simulink model "pe_marine_electrical_system"  (R2018b)
settings: Solver=ode23t  StartTime=0.0  StopTime=70  MaxStep=1e-3  RelTol=1e-3  AbsTol=1e-3
undefined symbols (not defined in the file): pe
libraries: fl_lib x41, pe_lib x25, nesl_utility x14, peSmAC1C x2, simulink x2
Description:
  | Marine Full Electric Propulsion Power System
  | 
  | This example shows a representative marine half-ship electrical power system with
  | base load, hotel load, bow thrusters and electric propulsion.
  | 
  | The principal components of the system are:
  | *) 30 MVA Gas Turbine, Round Rotor Alternator
  | *) 5 MVA Diesel Generator, Salient Pole Alternator
  | *) 11.5 MVA Base Load
  | *) 6 MVA Switched Hotel Load
  | *) 20 MVA Average-Value Propulsion Rectifier
  | *) 1 MVA Direct Online Start, Squirrel Cage Bow Thrusters
  | 
  | The sequence of events during the simulation is:
  | *) 10 seconds - Hotel Load disconnected
  | *) 20 seconds - Propulsion begins ramping up
  | *) 30 seconds - Full power ahead
  | *) 40 seconds - Propulsion begins ramping down
  | *) 50 seconds - Bow Thrusters start up
  | *) 60 seconds - Hotel Load connected
  | 
  | To view full results, run the simulation, and enter at the MATLAB command
  | prompt: sscexplore(pe_marine_electrical_system_simlog)
  | 
  | Copyright 2014-2017 The MathWorks, Inc.
settings Model: Creator=The MathWorks, Inc.  LastModifiedBy=hood000j
settings SolverCC: AutoScaleAbsTol=off  MaxConsecutiveMinStep=5
settings DataIOCC: LimitDataPoints=on  SaveFormat=Array
settings OptimizationCC: BlockReduction=off  BooleanDataType=off  LifeSpan=inf
settings DebuggingCC: SaveWithParameterizedLinksMsg=none  UnderspecifiedInitializationDetection=Classic  MergeDetectMultiDrivingBlocksExec=none  SignalResolutionControl=TryResolveAllWithWarning  AllowSymbolicDim=off  LibraryContextMissingDiagnostic=none  StrictBusMsg=ErrorOnBusTreatedAsVector  SFUnexpectedBacktrackingDiag=warning  SFNoUnconditionalDefaultTransitionDiag=warning  SFExecutionAtInitializationDiag=none
settings HardwareCC: ProdBitPerPointer=32  ProdBitPerSizeT=32  ProdBitPerPtrDiffT=32  ProdLargestAtomicFloat=None  ProdIntDivRoundTo=Undefined  ProdEndianess=Unspecified  ProdWordSize=32  ProdHWDeviceType=32-bit Generic  TargetUnknown=on
settings ModelReferenceCC: PropagateSignalLabelsOutOfModel=off
settings SFSimCC: SimUseLocalCustomCode=off
settings RTWCC: RTWUseLocalCustomCode=off
settings CodeAppCC: StateflowObjectComments=on
settings GRTTargetCC: TargetLangStandard=C89/C90 (ANSI)  GeneratePreprocessorConditionals=Disable all
settings ConfigComp: CovMetricSettings=dw  CovHtmlReporting=on  CovSaveCumulativeToWorkspaceVar=on  CovSaveSingleToWorkspaceVar=on  CovExternalEMLEnable=off  CovSFcnEnable=off
settings SimscapeCC: SimscapeLogType=local  SimscapeLogName=pe_marine_electrical_system_simlog  SimscapeLogLimitData=off

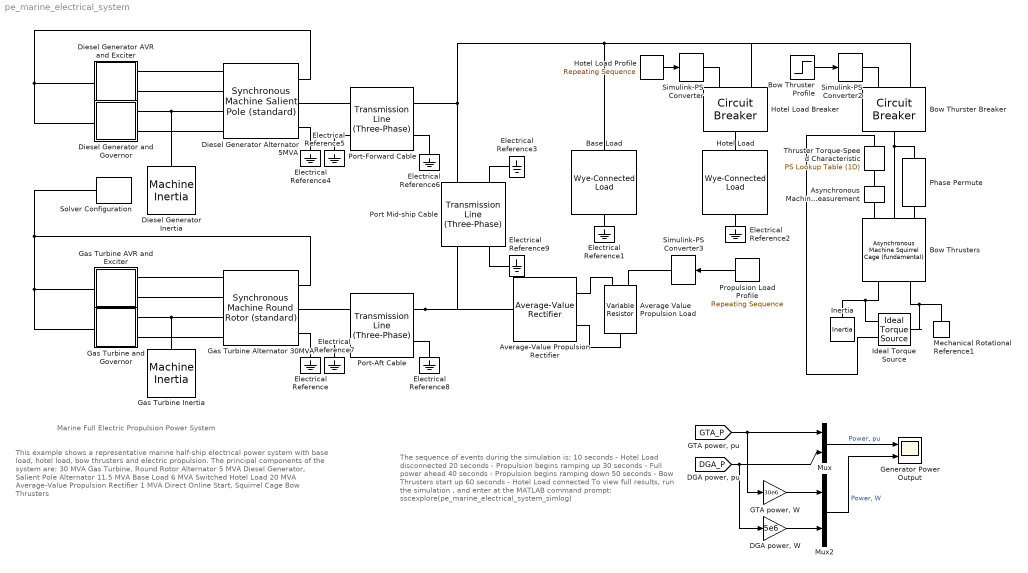
== system pe_marine_electrical_system ==
  note: The sequence of events during the simulation is:
      | 10 seconds - Hotel Load disconnected
      | 20 seconds - Propulsion begins ramping up
      | 30 seconds - Full power ahead
      | 40 seconds - Propulsion begins ramping down
      | 50 seconds - Bow Thrusters start up
      | 60 seconds - Hotel Load connected
      | To view full results, run the simulation , and enter at the MATLAB command
      | prompt: sscexplore(pe_marine_electrical_system_simlog)
  note: Marine Full Electric Propulsion Power System
  note: This example shows a representative marine half-ship electrical power system with
      | base load, hotel load, bow thrusters and electric propulsion.
      | The principal components of the system are:
      | 30 MVA Gas Turbine, Round Rotor Alternator
      | 5 MVA Diesel Generator, Salient Pole Alternator
      | 11.5 MVA Base Load
      | 6 MVA Switched Hotel Load
      | 20 MVA Average-Value Propulsion Rectifier
      | 1 MVA Direct Online Start, Squirrel Cage Bow Thrusters
  Asynchronous Machine Measurement : pe_lib/Machines/Asynchronous Machine Measurement  output_idx=2
      settings: SourceProductName=Simscape Power Systems  SourceProductBaseCode=PS  LogSimulationData=on
  Average Value Propulsion Load : fl_lib/Electrical/Electrical Elements/Variable Resistor  Rmin=0 Ohm  i_specify=off  i_priority=High  i=0 A  i_nominal_specify=off  i_nominal_unit=A  i_nominal_value=1  v_specify=off  v_priority=High  v=0 V  v_nominal_specify=off  v_nominal_unit=V  v_nominal_value=1
      settings: LogSimulationData=on
  Average-Value Propulsion Rectifier : pe_lib/Semiconductors/Average-Value Rectifier  VRated=4160 V  Pfixed=50e3 W
      settings: SourceProductName=Simscape Power Systems  SourceProductBaseCode=PS  LogSimulationData=on
  Base Load : pe_lib/Passive Devices/Wye-Connected Load  parameterization=2  component_structure=1  component_structure_PQ=4  R=1 Ohm  L=0.001 H  C=1e-6 F  IL0=[ 0 0 0 ] A  VC0=[ 0 0 0 ] V  R_parasitic=1e-6 Ohm  G_parasitic=1e-6 1/Ohm  VRated=4160 V  FRated=60 Hz  P=11.5e6 W  Qpos=700e3 V*A  Qneg=-100 V*A  Vmag0=4160 V  Vang0=0 deg  Freq0=60 Hz  R_parasitic_PQ=1e-6 Ohm  G_parasitic_PQ=1e-6 1/Ohm
      settings: SourceProductName=Simscape Power Systems  SourceProductBaseCode=PS  LogSimulationData=on
  Bow Thruster Profile : Step  Time=50  Before=1  After=0  SampleTime=0
  Bow Thrusters : pe_lib/Machines/Asynchronous Machine (Squirrel Cage)/Asynchronous Machine Squirrel Cage (fundamental)  SRated=1e6 V*A  VRated=4160 V  FRated=60 Hz  nPolePairs=5  squirrel_cage=pe.machines.asm_squirrel_cage.squirrelcage.Single  zero_sequence=pe.enum.park.zerosequence.include  Rs=0.0258  Lls=0.0930  Rrd=0.0145  Llrd=0.0424  Rrd1=0.0290  Llrd1=0.0848  Rrd2=0.0290  Llrd2=0.0848  Lm=1.7562  L0=0.0930  saturation_option=0  saturation_i=[0, .176, .396, .792, 1.1, 1.496, 2.2, 2.992, 4.18, 5.28]  saturation_v=[0, .2309, .4041, .5196, .5774, .6351, .6928, .7506, .8083, .866]  connection_option=int32(pe.Connection.delta)  param_option=pe.Parameterization.pu  angular_position_specify=off  angular_position_priority=None  angular_position=0 deg  angular_position_nominal_specify=off  angular_position_nominal_unit=deg  angular_position_nominal_value=1  pu_psids_specify=off  pu_psids_priority=None  pu_psids=0  pu_psids_nominal_specify=off  pu_psids_nominal_unit=1  pu_psids_nominal_value=1  pu_psiqs_specify=off  pu_psiqs_priority=None  pu_psiqs=0  pu_psiqs_nominal_specify=off  pu_psiqs_nominal_unit=1  pu_psiqs_nominal_value=1  pu_psi0s_specify=off  pu_psi0s_priority=None  pu_psi0s=0  pu_psi0s_nominal_specify=off  pu_psi0s_nominal_unit=1  pu_psi0s_nominal_value=1
      settings: SourceProductName=Simscape Power Systems  SourceProductBaseCode=PS  LogSimulationData=on
  Bow Thurster Breaker : pe_lib/Switches & Breakers/Circuit Breaker  R_closed=0.001 Ohm  G_open=1e-4 1/Ohm  threshold=0.5 V
      settings: SourceProductName=Simscape Power Systems  SourceProductBaseCode=PS  LogSimulationData=on
  "DGA power, W" : Gain  Gain=5e6
  Diesel Generator AVR and Exciter : Subsystem
  Diesel Generator Alternator 5MVA : pe_lib/Machines/Synchronous Machine (Salient Pole)/Synchronous Machine Salient Pole (standard)  SRated=5e6 V*A  VRated=4160 V  FRated=60 Hz  nPolePairs=4  fieldCircuitParameterization_option=2  baseEfd=216.54 V  baseIfd=50 A  zero_sequence=pe.enum.park.zerosequence.include  Ra=0.011  Xl=0.15  Xd=1.05  Xq=0.7  X0=0.15  Xdd=0.35  Xddd=0.25  Xqdd=0.325  d_option=1  Td0d=5.25 s  Tdd=1.75 s  Td0dd=0.03 s  Tddd=0.0214 s  q_option=1  Tq0dd=0.05 s  Tqdd=0.0232 s  saturation_option=0  axes_param=pe.enum.rotorangle.daxis  saturation_ifd=[0.00, 0.48, 0.76, 1.38, 1.79]  saturation_Vag=[0.00, 0.43, 0.59, 0.71, 0.76]  initialization_option=2  angular_position0=0 deg  pu_psid0=0  pu_psiq0=0  pu_psi00=0  pu_psifd0=0  pu_psi1d0=0  pu_psi1q0=0  Vmag0=4160 V  Vang0=0 deg  Pt0=2.5e6 V*A  Qt0=100e3 V*A  connection_option=int32(pe.Connection.wye)  num_q_dampers=1  rotor_offset=-pi / 2 rad  Xmin=1e-9
      settings: SourceProductName=Simscape Power Systems  SourceProductBaseCode=PS  LogSimulationData=on
  Diesel Generator Inertia : pe_lib/Machines/Machine Inertia  SRated=5e6 V*A  FRated=60 Hz  nPolePairs=4  inertia_option=2  J=27548 kg*m^2  H=3.525 s*W/V/A  damper_option=2  D=39.0509 N*m/(rad/s)  pu_D=0.01  initialization_option=2  fMechanical0=60 Hz  fElectrical0=60 Hz
      settings: SourceProductName=Simscape Power Systems  SourceProductBaseCode=PS  LogSimulationData=on
  Diesel Generator and Governor : Subsystem  mask(Governor and Prime Mover){pu_speed_reference=0.998, droop_percentage=5, pu_load_reference_setpoint=0.5, T_G=0.2, T_DG=0.3, base_torque=53051.6, pu_torque0=0.502754}
      mask prompts: pu_speed_reference "Speed reference, (pu)"; droop_percentage "Percentage droop, (%)"; pu_load_reference_setpoint "Load reference setpoint, (pu)"; T_G "Time constant of governor, (s)"; T_DG "Time constant of diesel generator, (s)"; base_torque "Base torque, (N*m)"; pu_torque0 "Initial torque, (pu)"
      mask help:
      | Implements a synchronous machine governor and prime mover. The prime mover is a diesel generator.
      |
      | The input to the block is a per-unit synchronous machine measurement vector.
      |
      | R and C are mechanical rotational ports.
  Electrical Reference{,1..9} (10 alike) : fl_lib/Electrical/Electrical Elements/Electrical Reference
  "GTA power, W" : Gain  Gain=30e6
  Gas Turbine AVR and Exciter : Subsystem
  Gas Turbine Inertia : pe_lib/Machines/Machine Inertia  SRated=30e6 V*A  FRated=60 Hz  nPolePairs=1  inertia_option=2  J=27548 kg*m^2  H=2.525 s*W/V/A  damper_option=2  D=39.0509 N*m/(rad/s)  pu_D=0.01  initialization_option=2  fMechanical0=60 Hz  fElectrical0=60 Hz
      settings: SourceProductName=Simscape Power Systems  SourceProductBaseCode=PS  LogSimulationData=on
  "Gas Turbine and Governor " : Subsystem  mask(Governor and Prime Mover){pu_speed_reference=0.998, droop_percentage=5, pu_load_reference_setpoint=0.5, T_G=0.1, T_GT=0.2, base_torque=79577.5, pu_torque0=0.500751}
      mask prompts: pu_speed_reference "Speed reference, (pu)"; droop_percentage "Percentage droop, (%)"; pu_load_reference_setpoint "Load reference setpoint, (pu)"; T_G "Time constant of governor, (s)"; T_GT "Time constant of gas turbine, (s)"; base_torque "Base torque, (N*m)"; pu_torque0 "Initial torque, (pu)"
      mask help:
      | Implements a synchronous machine governor and prime mover. The prime mover is a gas turbine.
      |
      | The input to the block is a per-unit synchronous machine measurement vector.
      |
      | R and C are mechanical rotational ports.
  Gas Turbine Alternator 30MVA : pe_lib/Machines/Synchronous Machine (Round Rotor)/Synchronous Machine Round Rotor (standard)  SRated=30e6 V*A  VRated=4160 V  FRated=60 Hz  nPolePairs=1  fieldCircuitParameterization_option=2  baseEfd=92.95 V  baseIfd=200 A  zero_sequence=pe.enum.park.zerosequence.include  Ra=0.003  Xl=0.15  Xd=1.81  Xq=1.76  X0=0.15  Xdd=0.3  Xqd=0.65  Xddd=0.23  Xqdd=0.25  d_option=1  Td0d=8 s  Tdd=1.3260 s  Td0dd=0.03 s  Tddd=0.0230 s  q_option=1  Tq0d=1 s  Tqd=0.3693 s  Tq0dd=0.07 s  Tqdd=0.0269 s  saturation_option=0  axes_param=pe.enum.rotorangle.daxis  saturation_ifd=[0.00, 0.48, 0.76, 1.38, 1.79]  saturation_Vag=[0.00, 0.80, 1.08, 1.31, 1.40]  initialization_option=2  angular_position0=0 deg  pu_psid0=0  pu_psiq0=0  pu_psi00=0  pu_psifd0=0  pu_psi1d0=0  pu_psi1q0=0  pu_psi2q0=0  Vmag0=4160 V  Vang0=0 deg  Pt0=15e6 V*A  Qt0=600e3 V*A  connection_option=int32(pe.Connection.wye)  num_q_dampers=2  rotor_offset=-pi / 2 rad  Xmin=1e-9
      settings: SourceProductName=Simscape Power Systems  SourceProductBaseCode=PS  LogSimulationData=on
  Generator Power Output : Scope  NumInputPorts=2
  Hotel Load : pe_lib/Passive Devices/Wye-Connected Load  parameterization=2  component_structure=1  component_structure_PQ=1  R=1 Ohm  L=0.001 H  C=1e-6 F  IL0=[ 0 0 0 ] A  VC0=[ 0 0 0 ] V  R_parasitic=1e-6 Ohm  G_parasitic=1e-6 1/Ohm  VRated=4160 V  FRated=60 Hz  P=6e6 W  Qpos=10e6 V*A  Qneg=-100 V*A  Vmag0=2.4e+4 V  Vang0=0 deg  Freq0=60 Hz  R_parasitic_PQ=1e-6 Ohm  G_parasitic_PQ=1e-6 1/Ohm
      settings: SourceProductName=Simscape Power Systems  SourceProductBaseCode=PS  LogSimulationData=on
  Hotel Load Breaker : pe_lib/Switches & Breakers/Circuit Breaker  R_closed=0.001 Ohm  G_open=1e-4 1/Ohm  threshold=0.5 V
      settings: SourceProductName=Simscape Power Systems  SourceProductBaseCode=PS  LogSimulationData=on
  Hotel Load Profile : simulink/Sources/Repeating Sequence  rep_seq_t=[0 9.99 10 59.9 60 100]  rep_seq_y=[0 0 1 1 0 0]
  Ideal Torque Source : fl_lib/Mechanical/Mechanical Sources/Ideal Torque Source
      settings: LogSimulationData=on
  Inertia : fl_lib/Mechanical/Rotational Elements/Inertia  inertia=1000 kg*m^2  w_specify=off  w_priority=High  w=0 rad/s  w_nominal_specify=off  w_nominal_unit=rad/s  w_nominal_value=1  t_specify=off  t_priority=High  t=0 N*m  t_nominal_specify=off  t_nominal_unit=N*m  t_nominal_value=1
      settings: LogSimulationData=on
  Mechanical Rotational Reference1 : fl_lib/Mechanical/Rotational Elements/Mechanical Rotational Reference
  Mux : Mux  Inputs=2
  Mux2 : Mux  Inputs=2
  Phase Permute : pe_lib/Connections/Phase Permute
      settings: SourceProductName=Simscape Power Systems  SourceProductBaseCode=PS  LogSimulationData=on
  Port Mid-ship Cable : pe_lib/Passive Devices/Transmission Line (Three-Phase)  length=0.2 km  R=0.02 Ohm/km  L=0.5 mH/km  M=0.1 mH/km  Cl=0.3 uF/km  Cg=0 uF/km  Rm=0 Ohm/km  N=1  R_parasitic=1e-6 Ohm  G_parasitic=1e-6 1/Ohm
      settings: SourceProductName=Simscape Power Systems  SourceProductBaseCode=PS  LogSimulationData=on
  Port-Aft Cable : pe_lib/Passive Devices/Transmission Line (Three-Phase)  length=0.1 km  R=0.02 Ohm/km  L=0.5 mH/km  M=0.1 mH/km  Cl=0.3 uF/km  Cg=0 uF/km  Rm=0 Ohm/km  N=1  R_parasitic=1e-6 Ohm  G_parasitic=1e-6 1/Ohm
      settings: SourceProductName=Simscape Power Systems  SourceProductBaseCode=PS  LogSimulationData=on
  Port-Forward Cable : pe_lib/Passive Devices/Transmission Line (Three-Phase)  length=0.1 km  R=0.02 Ohm/km  L=0.5 mH/km  M=0.1 mH/km  Cl=0.3 uF/km  Cg=0 uF/km  Rm=0 Ohm/km  N=1  R_parasitic=1e-6 Ohm  G_parasitic=1e-6 1/Ohm
      settings: SourceProductName=Simscape Power Systems  SourceProductBaseCode=PS  LogSimulationData=on
  Propulsion Load Profile : simulink/Sources/Repeating Sequence  rep_seq_t=[0 20 27 30 40 43 50 100]  rep_seq_y=[100 100 10 2 2 10 100 100]
  Simulink-PS Converter : nesl_utility/Simulink-PS Converter  PhysicalDomain=network_engine_domain  SubClassName=ps_input  LeftPortType=input  RightPortType=output  PseudoPeriodic=off  Frequencies=[]  NoiseDistribution=none  NoiseParameters=[]  Unit=1  AffineConversion=off  FilteringAndDerivatives=zero  SimscapeFilterOrder=1  InputFilterTimeConstant=0.001  UdotUserProvided=1
  Simulink-PS Converter2 : nesl_utility/Simulink-PS Converter  PhysicalDomain=network_engine_domain  SubClassName=ps_input  LeftPortType=input  RightPortType=output  PseudoPeriodic=off  Frequencies=[]  NoiseDistribution=none  NoiseParameters=[]  Unit=1  AffineConversion=off  FilteringAndDerivatives=zero  SimscapeFilterOrder=1  InputFilterTimeConstant=0.001  UdotUserProvided=1
  Simulink-PS Converter3 : nesl_utility/Simulink-PS Converter  PhysicalDomain=network_engine_domain  SubClassName=ps_input  LeftPortType=input  RightPortType=output  PseudoPeriodic=off  Frequencies=[]  NoiseDistribution=none  NoiseParameters=[]  Unit=1  AffineConversion=off  FilteringAndDerivatives=zero  SimscapeFilterOrder=1  InputFilterTimeConstant=0.001  UdotUserProvided=1
  Solver Configuration : nesl_utility/Solver Configuration  PhysicalDomain=network_engine_domain  SubClassName=solver  LeftPortType=input  RightPortType=generic  Tones=[]  Harmonics=[]  SimulateNoise=off  Profile=off  UseLocalSampling=off  EnableSwitchedLinearOptims=on  FrequencyDomain=off  UseCCode=off  RelTol=0.001  AbsTol=1e-06  MinStep=1e-09  ToWorkspace=off  RevertToSquareIcSolve=off  NumHomotopyIterations=100  PhasorMode=off  PhasorModeNumHarmonics=1  DoDC=off  ResidualTolerance=1e-09  UseLocalSolver=on  LocalSolverChoice=NE_BACKWARD_EULER_ADVANCER  LocalSolverSampleTime=1e-3  DoFixedCost=on  MaxNonlinIter=3  MaxModeIter=2  LinearAlgebra=auto  EquationFormulation=NE_TIME_EF  DelaysMemoryBudget=1024  AutomaticFiltering=on  FilteringTimeConstant=0.001  PartitionStorageMethod=AS_NEEDED  PartitionMemoryBudget=1024
  Thruster Torque-Speed Characteristic : fl_lib/Physical Signals/Lookup Tables/PS Lookup Table (1D)  x=[0:0.1:2]  f=13262.9.*[0:0.1:2].^2  interp_method=2  extrap_method=1
      settings: SourceProductName=Simscape  SourceProductBaseCode=SS  LogSimulationData=on
  wires:
  Hotel Load Profile/1 -> Simulink-PS Converter/1
  Bow Thruster Profile/1 -> Simulink-PS Converter2/1
  Propulsion Load Profile/1 -> Simulink-PS Converter3/1
  [GTA_P] -> Mux/1, "GTA power, W"/1
  [DGA_P] -> Mux/2, "DGA power, W"/1
  Mux/1 -> Generator Power Output/1  "Power, pu"
  "GTA power, W"/1 -> Mux2/1
  "DGA power, W"/1 -> Mux2/2
  Mux2/1 -> Generator Power Output/2  "Power, W"
  connections:
  Electrical Reference1/LConn1 -- Base Load/RConn1
  Port-Aft Cable/RConn1 -- Port Mid-ship Cable/RConn1 -- Average-Value Propulsion Rectifier/LConn1
  Gas Turbine AVR and Exciter/RConn1 -- Gas Turbine Alternator 30MVA/LConn1
  Gas Turbine Alternator 30MVA/RConn1 -- "Gas Turbine and Governor "/LConn1 -- Gas Turbine AVR and Exciter/LConn1 -- Solver Configuration/RConn1
  Gas Turbine AVR and Exciter/RConn2 -- Gas Turbine Alternator 30MVA/LConn2
  Gas Turbine Alternator 30MVA/RConn3 -- Electrical Reference/LConn1
  "Gas Turbine and Governor "/RConn2 -- Gas Turbine Alternator 30MVA/LConn4
  "Gas Turbine and Governor "/RConn1 -- Gas Turbine Inertia/LConn1 -- Gas Turbine Alternator 30MVA/LConn3
  Electrical Reference2/LConn1 -- Hotel Load/RConn1
  Hotel Load Breaker/RConn1 -- Hotel Load/LConn1
  Simulink-PS Converter/RConn1 -- Hotel Load Breaker/LConn1
  Diesel Generator and Governor/LConn1 -- Diesel Generator Alternator 5MVA/RConn1 -- Diesel Generator AVR and Exciter/LConn1
  Diesel Generator and Governor/RConn1 -- Diesel Generator Alternator 5MVA/LConn3 -- Diesel Generator Inertia/LConn1
  Diesel Generator Alternator 5MVA/LConn4 -- Diesel Generator and Governor/RConn2
  Diesel Generator Alternator 5MVA/RConn3 -- Electrical Reference4/LConn1
  Diesel Generator Alternator 5MVA/LConn2 -- Diesel Generator AVR and Exciter/RConn2
  Diesel Generator Alternator 5MVA/LConn1 -- Diesel Generator AVR and Exciter/RConn1
  Diesel Generator Alternator 5MVA/RConn2 -- Port-Forward Cable/LConn1
  Electrical Reference5/LConn1 -- Port-Forward Cable/LConn2
  Port-Forward Cable/RConn2 -- Electrical Reference6/LConn1
  Port-Aft Cable/LConn1 -- Gas Turbine Alternator 30MVA/RConn2
  Electrical Reference7/LConn1 -- Port-Aft Cable/LConn2
  Port-Aft Cable/RConn2 -- Electrical Reference8/LConn1
  Simulink-PS Converter2/RConn1 -- Bow Thurster Breaker/LConn1
  Bow Thrusters/RConn2 -- Phase Permute/LConn1 -- Bow Thurster Breaker/RConn1
  Bow Thrusters/LConn2 -- Ideal Torque Source/LConn1 -- Mechanical Rotational Reference1/LConn1
  Inertia/LConn1 -- Ideal Torque Source/RConn2 -- Bow Thrusters/LConn1
  Phase Permute/RConn1 -- Bow Thrusters/RConn3
  Average-Value Propulsion Rectifier/RConn1 -- Average Value Propulsion Load/LConn2
  Average-Value Propulsion Rectifier/RConn2 -- Average Value Propulsion Load/RConn1
  Simulink-PS Converter3/RConn1 -- Average Value Propulsion Load/LConn1
  Electrical Reference3/LConn1 -- Port Mid-ship Cable/LConn2
  Electrical Reference9/LConn1 -- Port Mid-ship Cable/RConn2
  Port-Forward Cable/RConn1 -- Base Load/LConn1 -- Bow Thurster Breaker/LConn2 -- Hotel Load Breaker/LConn2 -- Port Mid-ship Cable/LConn1
  Thruster Torque-Speed Characteristic/LConn1 -- Asynchronous Machine Measurement/RConn1
  Asynchronous Machine Measurement/LConn1 -- Bow Thrusters/RConn1
  Thruster Torque-Speed Characteristic/RConn1 -- Ideal Torque Source/RConn1

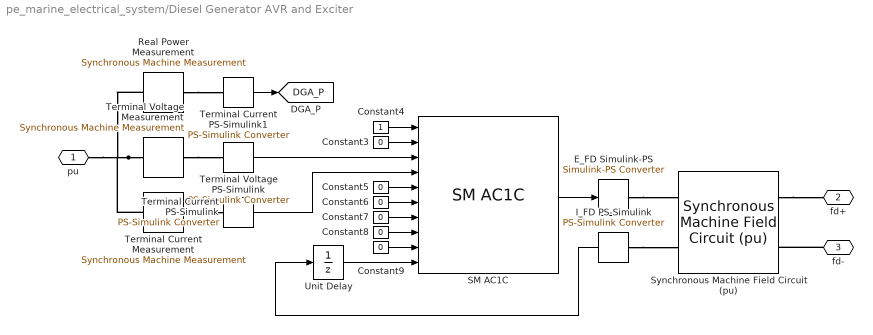
== system pe_marine_electrical_system/Diesel Generator AVR and Exciter ==
  Constant{3,5..9} (6 alike) : Constant  Value=0
  Constant4 : Constant
  "E_FD Simulink-PS " : nesl_utility/Simulink-PS Converter  PhysicalDomain=network_engine_domain  SubClassName=ps_input  LeftPortType=input  RightPortType=output  PseudoPeriodic=off  Frequencies=[]  NoiseDistribution=none  NoiseParameters=[]  Unit=1  AffineConversion=off  FilteringAndDerivatives=provide  SimscapeFilterOrder=1  InputFilterTimeConstant=.001  UdotUserProvided=0
  I_FD PS-Simulink : nesl_utility/PS-Simulink Converter  PhysicalDomain=network_engine_domain  SubClassName=ps_output  LeftPortType=input  RightPortType=output  PseudoPeriodic=off  Frequencies=[]  Unit=1  AffineConversion=off
  Real Power Measurement : pe_lib/Machines/Synchronous Machine Measurement  output_idx=12
      settings: SourceProductName=Simscape Power Systems  SourceProductBaseCode=PS  LogSimulationData=on
  SM AC1C : peSmAC1C/SM AC1C  E_FD0=1.14125  Ts=-1  R_C=0  X_C=0  T_R=0  K_A=400  T_A=0.02  T_B=0  T_C=0  K_F=0.03  T_F=1  V_Amax=14.5  V_Amin=-14.5  E_FEmax=6.03  E_FEmin=-5.43  oelInputLocation=Unused  uelInputLocation=Unused  sclInputLocation=Unused  K_E=1  T_E=0.8  K_C=0.2  K_D=0.38  E_1=4.18  S_E_E1=0.1  E_2=3.14  S_E_E2=0.03
  Synchronous Machine Field Circuit (pu) : pe_lib/Machines/Synchronous Machine Field Circuit (pu)  SRated=5e6 V*A  FRated=60 Hz  fieldCircuitParameterization_option=2  baseEfd=92.95 V  baseIfd=50 A  parameterization_option=2  Ladu=1.66  Rfd=0.0006  Xl=0.15  Xd=1.05  Xdd=0.35  Xddd=0.23  d_option=pe.enum.circuit.open  Td0d=5.25 s  Tdd=1.3260 s  Td0dd=0.03 s  Tddd=0.0230 s
      settings: SourceProductName=Simscape Power Systems  SourceProductBaseCode=PS  LogSimulationData=on
  Terminal Current Measurement : pe_lib/Machines/Synchronous Machine Measurement  output_idx=15
      settings: SourceProductName=Simscape Power Systems  SourceProductBaseCode=PS  LogSimulationData=on
  Terminal Current PS-Simulink : nesl_utility/PS-Simulink Converter  PhysicalDomain=network_engine_domain  SubClassName=ps_output  LeftPortType=input  RightPortType=output  PseudoPeriodic=off  Frequencies=[]  Unit=1  AffineConversion=off
  Terminal Current PS-Simulink1 : nesl_utility/PS-Simulink Converter  PhysicalDomain=network_engine_domain  SubClassName=ps_output  LeftPortType=input  RightPortType=output  PseudoPeriodic=off  Frequencies=[]  Unit=1  AffineConversion=off
  Terminal Voltage Measurement : pe_lib/Machines/Synchronous Machine Measurement  output_idx=14
      settings: SourceProductName=Simscape Power Systems  SourceProductBaseCode=PS  LogSimulationData=on
  Terminal Voltage PS-Simulink : nesl_utility/PS-Simulink Converter  PhysicalDomain=network_engine_domain  SubClassName=ps_output  LeftPortType=input  RightPortType=output  PseudoPeriodic=off  Frequencies=[]  Unit=1  AffineConversion=off
  Unit Delay : UnitDelay  InitialCondition=1.14125  SampleTime=-1
  pu : PMIOPort  Side=Left
  fd+ : PMIOPort  Port=2  Side=Right
  fd- : PMIOPort  Port=3  Side=Right
  tag scope: DGA_P=global
  wires:
  Terminal Current PS-Simulink1/1 -> [DGA_P]
  Constant6/1 -> SM AC1C/6
  Terminal Voltage PS-Simulink/1 -> SM AC1C/3
  Terminal Current PS-Simulink/1 -> SM AC1C/4
  Constant7/1 -> SM AC1C/7
  I_FD PS-Simulink/1 -> Unit Delay/1
  SM AC1C/1 -> "E_FD Simulink-PS "/1
  Constant9/1 -> SM AC1C/9
  Constant8/1 -> SM AC1C/8
  Constant4/1 -> SM AC1C/1
  Constant3/1 -> SM AC1C/2
  Unit Delay/1 -> SM AC1C/10
  Constant5/1 -> SM AC1C/5
  connections:
  fd-/RConn1 -- Synchronous Machine Field Circuit (pu)/RConn2
  Synchronous Machine Field Circuit (pu)/RConn1 -- fd+/RConn1
  I_FD PS-Simulink/LConn1 -- Synchronous Machine Field Circuit (pu)/LConn2
  "E_FD Simulink-PS "/RConn1 -- Synchronous Machine Field Circuit (pu)/LConn1
  Terminal Voltage Measurement/LConn1 -- Terminal Current Measurement/LConn1 -- Real Power Measurement/LConn1 -- pu/RConn1
  Terminal Voltage Measurement/RConn1 -- Terminal Voltage PS-Simulink/LConn1
  Terminal Current Measurement/RConn1 -- Terminal Current PS-Simulink/LConn1
  Real Power Measurement/RConn1 -- Terminal Current PS-Simulink1/LConn1

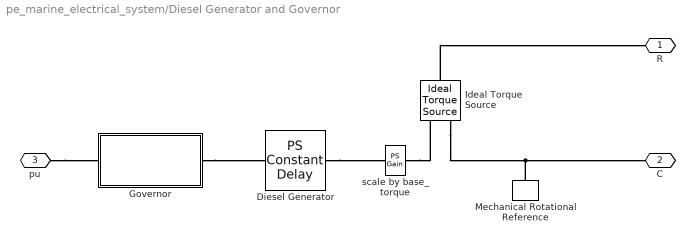
== system pe_marine_electrical_system/Diesel Generator and Governor ==
  Diesel Generator : fl_lib/Physical Signals/Delays/PS Constant Delay  InputHistory=pu_torque0  DelayTime=T_DG s
      settings: SourceProductName=Simscape  SourceProductBaseCode=SS
  Governor : Subsystem
  Ideal Torque Source : fl_lib/Mechanical/Mechanical Sources/Ideal Torque Source
  Mechanical Rotational Reference : fl_lib/Mechanical/Rotational Elements/Mechanical Rotational Reference
  scale by base_torque : fl_lib/Physical Signals/Functions/PS Gain  gain=base_torque
  R : PMIOPort  Side=Right
  C : PMIOPort  Port=2  Side=Right
  pu : PMIOPort  Port=3  Side=Left
  connections:
  Diesel Generator/RConn1 -- scale by base_torque/LConn1
  scale by base_torque/RConn1 -- Ideal Torque Source/RConn1
  pu/RConn1 -- Governor/LConn1
  Governor/RConn1 -- Diesel Generator/LConn1
  Ideal Torque Source/LConn1 -- R/RConn1
  Mechanical Rotational Reference/LConn1 -- Ideal Torque Source/RConn2 -- C/RConn1

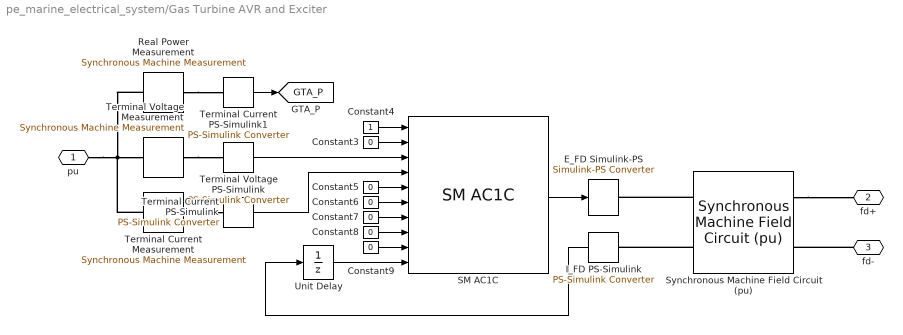
== system pe_marine_electrical_system/Gas Turbine AVR and Exciter ==
  Constant{3,5..9} (6 alike) : Constant  Value=0
  Constant4 : Constant
  "E_FD Simulink-PS " : nesl_utility/Simulink-PS Converter  PhysicalDomain=network_engine_domain  SubClassName=ps_input  LeftPortType=input  RightPortType=output  PseudoPeriodic=off  Frequencies=[]  NoiseDistribution=none  NoiseParameters=[]  Unit=1  AffineConversion=off  FilteringAndDerivatives=provide  SimscapeFilterOrder=1  InputFilterTimeConstant=.001  UdotUserProvided=0
  I_FD PS-Simulink : nesl_utility/PS-Simulink Converter  PhysicalDomain=network_engine_domain  SubClassName=ps_output  LeftPortType=input  RightPortType=output  PseudoPeriodic=off  Frequencies=[]  Unit=1  AffineConversion=off
  Real Power Measurement : pe_lib/Machines/Synchronous Machine Measurement  output_idx=12
      settings: SourceProductName=Simscape Power Systems  SourceProductBaseCode=PS  LogSimulationData=on
  SM AC1C : peSmAC1C/SM AC1C  E_FD0=1.37673  Ts=-1  R_C=0  X_C=0  T_R=0  K_A=400  T_A=0.02  T_B=0  T_C=0  K_F=0.03  T_F=1  V_Amax=14.5  V_Amin=-14.5  E_FEmax=6.03  E_FEmin=-5.43  oelInputLocation=Unused  uelInputLocation=Unused  sclInputLocation=Unused  K_E=1  T_E=0.8  K_C=0.2  K_D=0.38  E_1=4.18  S_E_E1=0.1  E_2=3.14  S_E_E2=0.03
  Synchronous Machine Field Circuit (pu) : pe_lib/Machines/Synchronous Machine Field Circuit (pu)  SRated=30e6 V*A  FRated=60 Hz  fieldCircuitParameterization_option=2  baseEfd=92.95 V  baseIfd=200 A  parameterization_option=2  Ladu=1.66  Rfd=0.0006  Xl=0.15  Xd=1.81  Xdd=0.3  Xddd=0.23  d_option=pe.enum.circuit.open  Td0d=8 s  Tdd=1.3260 s  Td0dd=0.03 s  Tddd=0.0230 s
      settings: SourceProductName=Simscape Power Systems  SourceProductBaseCode=PS  LogSimulationData=on
  Terminal Current Measurement : pe_lib/Machines/Synchronous Machine Measurement  output_idx=15
      settings: SourceProductName=Simscape Power Systems  SourceProductBaseCode=PS  LogSimulationData=on
  Terminal Current PS-Simulink : nesl_utility/PS-Simulink Converter  PhysicalDomain=network_engine_domain  SubClassName=ps_output  LeftPortType=input  RightPortType=output  PseudoPeriodic=off  Frequencies=[]  Unit=1  AffineConversion=off
  Terminal Current PS-Simulink1 : nesl_utility/PS-Simulink Converter  PhysicalDomain=network_engine_domain  SubClassName=ps_output  LeftPortType=input  RightPortType=output  PseudoPeriodic=off  Frequencies=[]  Unit=1  AffineConversion=off
  Terminal Voltage Measurement : pe_lib/Machines/Synchronous Machine Measurement  output_idx=14
      settings: SourceProductName=Simscape Power Systems  SourceProductBaseCode=PS  LogSimulationData=on
  Terminal Voltage PS-Simulink : nesl_utility/PS-Simulink Converter  PhysicalDomain=network_engine_domain  SubClassName=ps_output  LeftPortType=input  RightPortType=output  PseudoPeriodic=off  Frequencies=[]  Unit=1  AffineConversion=off
  Unit Delay : UnitDelay  InitialCondition=1.37673  SampleTime=-1
  pu : PMIOPort  Side=Left
  fd+ : PMIOPort  Port=2  Side=Right
  fd- : PMIOPort  Port=3  Side=Right
  tag scope: GTA_P=global
  wires:
  Terminal Current PS-Simulink1/1 -> [GTA_P]
  Constant5/1 -> SM AC1C/5
  Constant4/1 -> SM AC1C/1
  Unit Delay/1 -> SM AC1C/10
  Constant3/1 -> SM AC1C/2
  Constant7/1 -> SM AC1C/7
  Constant9/1 -> SM AC1C/9
  I_FD PS-Simulink/1 -> Unit Delay/1
  Constant6/1 -> SM AC1C/6
  Constant8/1 -> SM AC1C/8
  Terminal Current PS-Simulink/1 -> SM AC1C/4
  Terminal Voltage PS-Simulink/1 -> SM AC1C/3
  SM AC1C/1 -> "E_FD Simulink-PS "/1
  connections:
  Terminal Current Measurement/RConn1 -- Terminal Current PS-Simulink/LConn1
  Terminal Voltage Measurement/RConn1 -- Terminal Voltage PS-Simulink/LConn1
  pu/RConn1 -- Terminal Current Measurement/LConn1 -- Real Power Measurement/LConn1 -- Terminal Voltage Measurement/LConn1
  Synchronous Machine Field Circuit (pu)/LConn1 -- "E_FD Simulink-PS "/RConn1
  Synchronous Machine Field Circuit (pu)/LConn2 -- I_FD PS-Simulink/LConn1
  Synchronous Machine Field Circuit (pu)/RConn1 -- fd+/RConn1
  fd-/RConn1 -- Synchronous Machine Field Circuit (pu)/RConn2
  Real Power Measurement/RConn1 -- Terminal Current PS-Simulink1/LConn1

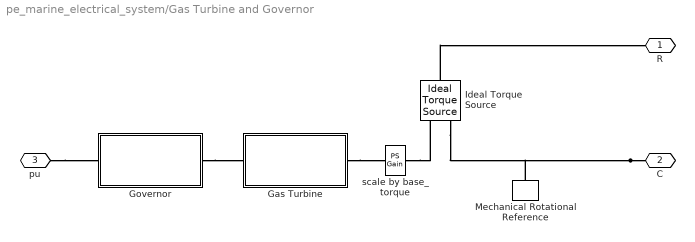
== system pe_marine_electrical_system/Gas Turbine and Governor  ==
  Gas Turbine : Subsystem
  Governor : Subsystem
  Ideal Torque Source : fl_lib/Mechanical/Mechanical Sources/Ideal Torque Source
  Mechanical Rotational Reference : fl_lib/Mechanical/Rotational Elements/Mechanical Rotational Reference
  scale by base_torque : fl_lib/Physical Signals/Functions/PS Gain  gain=base_torque
  R : PMIOPort  Side=Right
  C : PMIOPort  Port=2  Side=Right
  pu : PMIOPort  Port=3  Side=Left
  connections:
  C/RConn1 -- Ideal Torque Source/RConn2 -- Mechanical Rotational Reference/LConn1
  Ideal Torque Source/LConn1 -- R/RConn1
  Governor/RConn1 -- Gas Turbine/LConn1
  pu/RConn1 -- Governor/LConn1
  scale by base_torque/RConn1 -- Ideal Torque Source/RConn1
  Gas Turbine/RConn1 -- scale by base_torque/LConn1

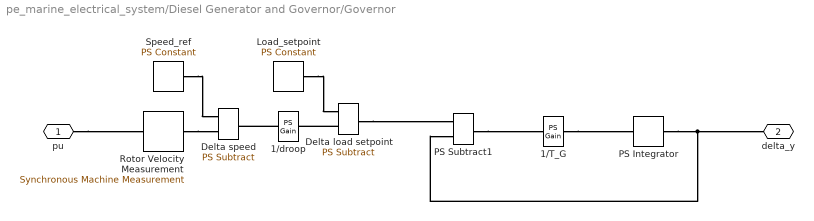
== system pe_marine_electrical_system/Diesel Generator and Governor/Governor ==
  1/T_G : fl_lib/Physical Signals/Functions/PS Gain  gain=1/T_G
  1/droop : fl_lib/Physical Signals/Functions/PS Gain  gain=1/(droop_percentage/100)
  Delta load setpoint : fl_lib/Physical Signals/Functions/PS Subtract
      settings: SourceProductName=Simscape
  Delta speed : fl_lib/Physical Signals/Functions/PS Subtract
      settings: SourceProductName=Simscape
  Load_setpoint : fl_lib/Physical Signals/Sources/PS Constant  constant=pu_load_reference_setpoint
  PS Integrator : fl_lib/Physical Signals/Linear Operators/PS Integrator  x0=pu_torque0
      settings: SourceProductName=Simscape  SourceProductBaseCode=SS
  PS Subtract1 : fl_lib/Physical Signals/Functions/PS Subtract
      settings: SourceProductName=Simscape
  Rotor Velocity Measurement : pe_lib/Machines/Synchronous Machine Measurement  output_idx=4
      settings: SourceProductName=Simscape Power Systems  SourceProductBaseCode=PS
  Speed_ref : fl_lib/Physical Signals/Sources/PS Constant  constant=pu_speed_reference
  pu : PMIOPort  Side=Left
  delta_y : PMIOPort  Port=2  Side=Right
  connections:
  pu/RConn1 -- Rotor Velocity Measurement/LConn1
  Delta load setpoint/RConn1 -- PS Subtract1/LConn1
  Delta load setpoint/LConn2 -- 1/droop/RConn1
  Rotor Velocity Measurement/RConn1 -- Delta speed/LConn1
  Speed_ref/RConn1 -- Delta speed/LConn2
  1/droop/LConn1 -- Delta speed/RConn1
  Load_setpoint/RConn1 -- Delta load setpoint/LConn1
  1/T_G/RConn1 -- PS Integrator/LConn1
  PS Subtract1/RConn1 -- 1/T_G/LConn1
  PS Integrator/RConn1 -- PS Subtract1/LConn2 -- delta_y/RConn1

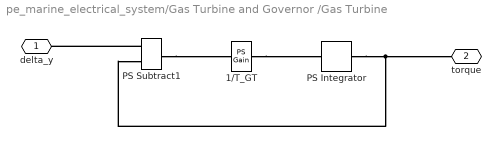
== system pe_marine_electrical_system/Gas Turbine and Governor /Gas Turbine ==
  1/T_GT : fl_lib/Physical Signals/Functions/PS Gain  gain=1/T_GT
  PS Integrator : fl_lib/Physical Signals/Linear Operators/PS Integrator  x0=pu_torque0
      settings: SourceProductName=Simscape  SourceProductBaseCode=SS
  PS Subtract1 : fl_lib/Physical Signals/Functions/PS Subtract
      settings: SourceProductName=Simscape
  delta_y : PMIOPort  Side=Left
  torque : PMIOPort  Port=2  Side=Right
  connections:
  1/T_GT/RConn1 -- PS Integrator/LConn1
  PS Subtract1/LConn1 -- delta_y/RConn1
  PS Subtract1/RConn1 -- 1/T_GT/LConn1
  PS Integrator/RConn1 -- PS Subtract1/LConn2 -- torque/RConn1

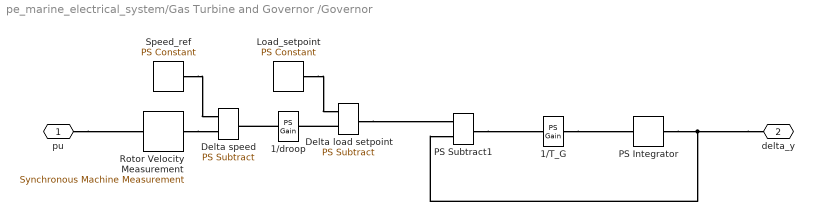
== system pe_marine_electrical_system/Gas Turbine and Governor /Governor ==
  1/T_G : fl_lib/Physical Signals/Functions/PS Gain  gain=1/T_G
  1/droop : fl_lib/Physical Signals/Functions/PS Gain  gain=1/(droop_percentage/100)
  Delta load setpoint : fl_lib/Physical Signals/Functions/PS Subtract
      settings: SourceProductName=Simscape
  Delta speed : fl_lib/Physical Signals/Functions/PS Subtract
      settings: SourceProductName=Simscape
  Load_setpoint : fl_lib/Physical Signals/Sources/PS Constant  constant=pu_load_reference_setpoint
  PS Integrator : fl_lib/Physical Signals/Linear Operators/PS Integrator  x0=pu_torque0
      settings: SourceProductName=Simscape  SourceProductBaseCode=SS
  PS Subtract1 : fl_lib/Physical Signals/Functions/PS Subtract
      settings: SourceProductName=Simscape
  Rotor Velocity Measurement : pe_lib/Machines/Synchronous Machine Measurement  output_idx=4
      settings: SourceProductName=Simscape Power Systems  SourceProductBaseCode=PS
  Speed_ref : fl_lib/Physical Signals/Sources/PS Constant  constant=pu_speed_reference
  pu : PMIOPort  Side=Left
  delta_y : PMIOPort  Port=2  Side=Right
  connections:
  delta_y/RConn1 -- PS Subtract1/LConn2 -- PS Integrator/RConn1
  PS Subtract1/RConn1 -- 1/T_G/LConn1
  1/T_G/RConn1 -- PS Integrator/LConn1
  Load_setpoint/RConn1 -- Delta load setpoint/LConn1
  1/droop/LConn1 -- Delta speed/RConn1
  Speed_ref/RConn1 -- Delta speed/LConn2
  Rotor Velocity Measurement/RConn1 -- Delta speed/LConn1
  Delta load setpoint/LConn2 -- 1/droop/RConn1
  Delta load setpoint/RConn1 -- PS Subtract1/LConn1
  pu/RConn1 -- Rotor Velocity Measurement/LConn1
